simulink subsystem "VehicleEOMRef"  (R2025a)
settings: Solver=VariableStepAuto  StartTime=0.0  StopTime=10.0  RelTol=1e-3
undefined symbols (not defined in the file): Accel_bIi, AngularMomentum, AngularMomentumDot, Asensed_bIb, Forces, Moments, Omeg_BIb, Omeg_BIb_IC, OmegDtI_BIb, Pos_bii, Pos_bii_IC, Q_i2b, Q_i2b_IC, SimIn, SimPar, StateStruct, Vel_bEb_IC, Vel_bIi
libraries: starslibMathOperations x38, starslibAxisTransformations x25, starslibAirData x8, starslibKinematicalEquations x5, starslibGeodesy x4
(part 1 of 2)
settings Model: Creator=drhill  LastModifiedBy=alhallmark
settings SolverCC: AlgebraicLoopSolver=TrustRegion
settings OptimizationCC: ReuseModelBlockBuffer=off
settings DebuggingCC: UnconnectedInputMsg=warning  UnconnectedOutputMsg=warning  UnconnectedLineMsg=warning
settings ModelReferenceCC: EnableRefExpFcnMdlSchedulingChecks=on
settings RTWCC: GPUComputeCapability=3.5  DLArmComputeVersion=19.05

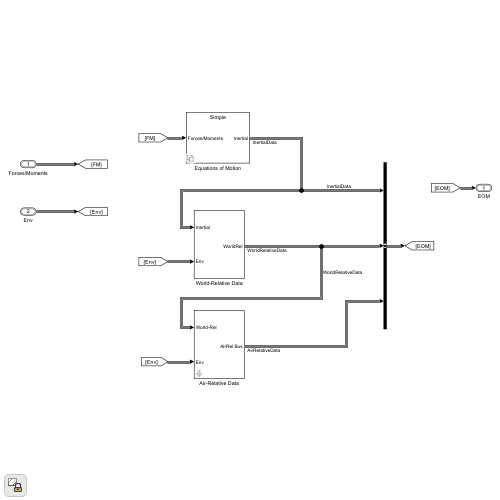
[thumbnail: Simulink's stored preview of the top-level diagram]
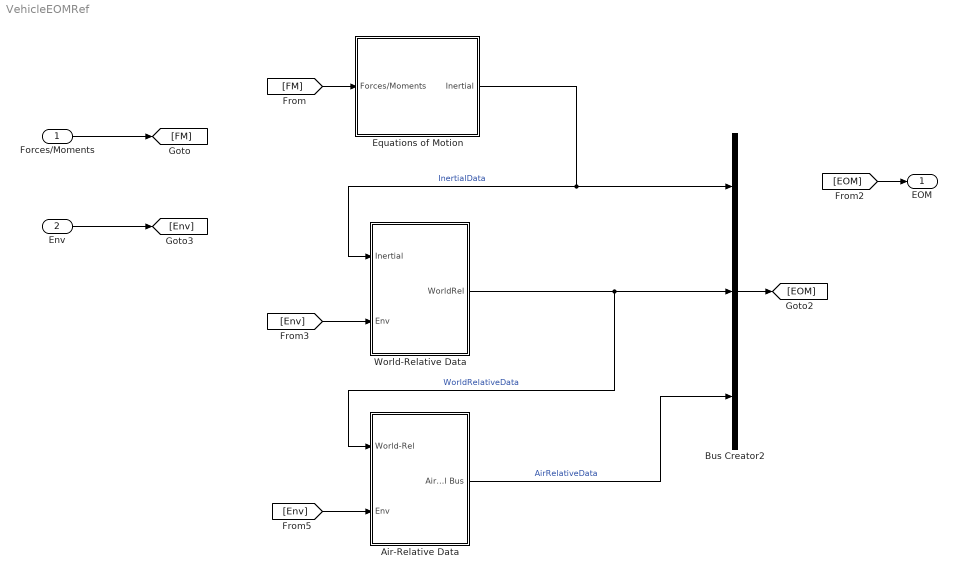
== system VehicleEOMRef ==
  Forces/Moments : Inport  OutDataTypeStr=Bus: ForceMomentBus
  Env : Inport  Port=2  OutDataTypeStr=Bus: EnvironmentBus
  Air-Relative Data : Subsystem  mask(Air-Relative Data (template)){}
      mask help: Template for common air-relative data.
  Bus Creator2 : BusCreator  Inputs=3  OutDataTypeStr=Bus: EomBus
  Equations of Motion : Subsystem  Variant=on  VariantControl=Variant1
  World-Relative Data : Subsystem
  EOM : Outport  OutDataTypeStr=Bus: EomBus
  wires:
  Forces/Moments/1 -> [FM]
  [FM] -> Equations of Motion/1(Forces/Moments)
  Bus Creator2/1 -> [EOM]
  [EOM] -> EOM/1
  Env/1 -> [Env]
  [Env] -> World-Relative Data/2(Env)
  [Env] -> Air-Relative Data/2(Env)
  Air-Relative Data/1(AirRel Bus) -> Bus Creator2/3  "AirRelativeData"
  Equations of Motion/1(Inertial) -> Bus Creator2/1, World-Relative Data/1(Inertial)  "InertialData"
  World-Relative Data/1(WorldRel) -> Air-Relative Data/1(World-Rel), Bus Creator2/2  "WorldRelativeData"

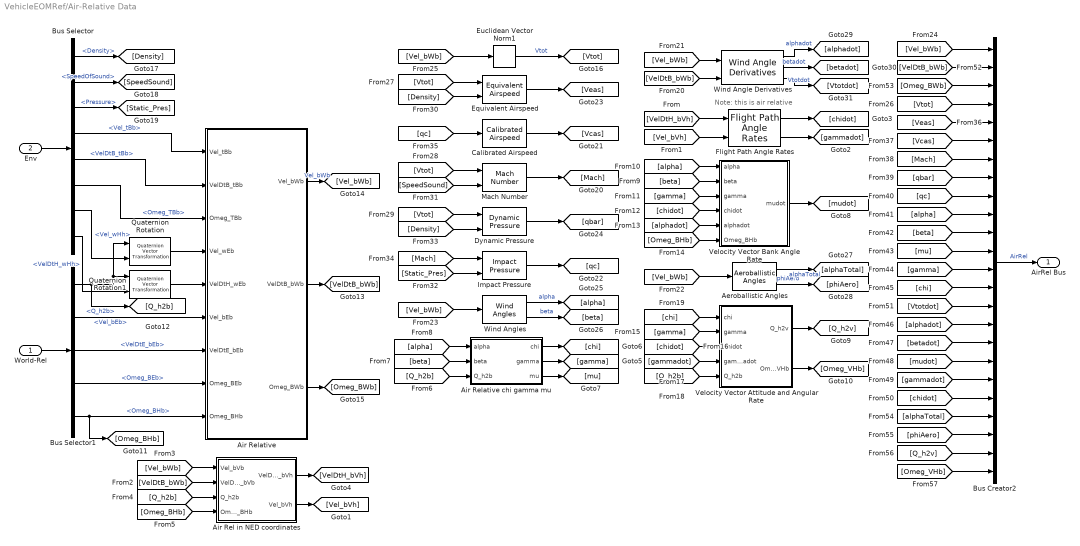
== system VehicleEOMRef/Air-Relative Data ==
  note: Note: this is air relative
  World-Rel : Inport
  Env : Inport  Port=2
  Aeroballistic Angles : starslibAirData/Aeroballistic Angles
  Air Rel in NED coordinates : Subsystem
  Air Relative : Subsystem
  Air Relative chi gamma mu : Subsystem
  Bus Creator2 : BusCreator  Inputs=24  OutDataTypeStr=Bus: AirRelBus
  Bus Selector : BusSelector  OutputSignals=Atmosphere.Density,Atmosphere.SpeedOfSound,Atmosphere.Pressure,Turbulence.Vel_tBb,Turbulence.VelDtB_tBb,Turbulence.Omeg_TBb,Wind.Vel_wHh,Wind.VelDtH_wHh
  Bus Selector1 : BusSelector  OutputSignals=Q_h2b,Vel_bEb,VelDtE_bEb,Omeg_BEb,Omeg_BHb
  Calibrated Airspeed : starslibAirData/Calibrated Airspeed  rhoref=SimIn.Environment.Atmos.rho0  Pref=SimIn.Environment.Atmos.Ps0  gamma=SimIn.Environment.Atmos.gamma
  Dynamic Pressure : starslibAirData/Dynamic Pressure
  Equivalent Airspeed : starslibAirData/Equivalent Airspeed  rhoref=SimIn.Environment.Atmos.rho0
  Euclidean Vector Norm1 : starslibMathOperations/Euclidean Vector Norm  dim=1
  Flight Path Angle Rates : starslibKinematicalEquations/Flight Path Angle Rates
  Impact Pressure : starslibAirData/Impact Pressure  gamma=SimIn.Environment.Atmos.gamma
  Mach Number : starslibAirData/Mach Number
  Quaternion Rotation : starslibAxisTransformations/Quaternion Vector Transformation  n=0
  Quaternion Rotation1 : starslibAxisTransformations/Quaternion Vector Transformation  n=0
  Velocity Vector Attitude and Angular Rate : Subsystem
  Velocity Vector Bank Angle Rate : Subsystem
  Wind Angle Derivatives : starslibAirData/Wind Angle Derivatives
  Wind Angles : starslibAirData/Wind Angles
  AirRel Bus : Outport
  wires:
  [Omeg_VHb] -> Bus Creator2/24
  [Q_h2v] -> Bus Creator2/23
  [phiAero] -> Bus Creator2/22
  [alphaTotal] -> Bus Creator2/21
  [Omeg_BWb] -> Bus Creator2/3
  [VelDtB_bWb] -> Bus Creator2/2
  [Vtotdot] -> Bus Creator2/15
  [chidot] -> Bus Creator2/20
  [gammadot] -> Bus Creator2/19
  [mudot] -> Bus Creator2/18
  [betadot] -> Bus Creator2/17
  [alphadot] -> Bus Creator2/16
  [chi] -> Bus Creator2/14
  [gamma] -> Bus Creator2/13
  [mu] -> Bus Creator2/12
  [beta] -> Bus Creator2/11
  [alpha] -> Bus Creator2/10
  [qc] -> Bus Creator2/9
  [qbar] -> Bus Creator2/8
  [Mach] -> Bus Creator2/7
  [Vcas] -> Bus Creator2/6
  [Veas] -> Bus Creator2/5
  Wind Angle Derivatives/3 -> [Vtotdot]  "Vtotdot"
  Wind Angle Derivatives/2 -> [betadot]  "betadot"
  Wind Angle Derivatives/1 -> [alphadot]  "alphadot"
  Aeroballistic Angles/2 -> [phiAero]  "phiAero"
  Aeroballistic Angles/1 -> [alphaTotal]  "alphaTotal"
  Wind Angles/2 -> [beta]  "beta"
  Wind Angles/1 -> [alpha]  "alpha"
  [qc] -> Calibrated Airspeed/1
  Calibrated Airspeed/1 -> [Vcas]
  [Mach] -> Impact Pressure/1
  Mach Number/1 -> [Mach]
  [Density] -> Dynamic Pressure/2
  [Density] -> Equivalent Airspeed/2
  [SpeedSound] -> Mach Number/2
  [Static_Pres] -> Impact Pressure/2
  [Vtot] -> Dynamic Pressure/1
  [Vtot] -> Mach Number/1
  [Vtot] -> Equivalent Airspeed/1
  Euclidean Vector Norm1/1 -> [Vtot]  "Vtot"
  Air Relative/3(Omeg_BWb) -> [Omeg_BWb]
  [Vel_bWb] -> Euclidean Vector Norm1/1
  [Vel_bWb] -> Bus Creator2/1
  [Vel_bWb] -> Wind Angles/1
  [Vel_bWb] -> Aeroballistic Angles/1
  [VelDtB_bWb] -> Wind Angle Derivatives/2
  [Vel_bWb] -> Wind Angle Derivatives/1
  Velocity Vector Attitude and Angular Rate/2(Omeg_VHb) -> [Omeg_VHb]
  Velocity Vector Attitude and Angular Rate/1(Q_h2v) -> [Q_h2v]
  [chi] -> Velocity Vector Attitude and Angular Rate/1(chi)
  [gammadot] -> Velocity Vector Attitude and Angular Rate/4(gammadot)
  [gamma] -> Velocity Vector Attitude and Angular Rate/2(gamma)
  [chidot] -> Velocity Vector Attitude and Angular Rate/3(" chidot")
  [Q_h2b] -> Velocity Vector Attitude and Angular Rate/5(Q_h2b)
  [Omeg_BHb] -> Velocity Vector Bank Angle Rate/6(Omeg_BHb)
  [alphadot] -> Velocity Vector Bank Angle Rate/5(alphadot)
  [chidot] -> Velocity Vector Bank Angle Rate/4(chidot)
  [gamma] -> Velocity Vector Bank Angle Rate/3(gamma)
  [alpha] -> Velocity Vector Bank Angle Rate/1(alpha)
  [beta] -> Velocity Vector Bank Angle Rate/2(beta)
  Velocity Vector Bank Angle Rate/1(mudot) -> [mudot]
  [alpha] -> Air Relative chi gamma mu/1(alpha)
  [beta] -> Air Relative chi gamma mu/2(beta)
  Air Relative chi gamma mu/3(mu) -> [mu]
  Air Relative chi gamma mu/2(gamma) -> [gamma]
  Air Relative chi gamma mu/1(chi) -> [chi]
  [Q_h2b] -> Air Relative chi gamma mu/3(Q_h2b)
  [Omeg_BHb] -> Air Rel in NED coordinates/4(Omeg_BHb)
  [Q_h2b] -> Air Rel in NED coordinates/3(Q_h2b)
  [Vel_bWb] -> Air Rel in NED coordinates/1(Vel_bVb)
  [VelDtB_bWb] -> Air Rel in NED coordinates/2(VelDtB_bVb)
  Air Rel in NED coordinates/2(Vel_bVh) -> [Vel_bVh]
  Air Rel in NED coordinates/1(VelDtH_bVh) -> [VelDtH_bVh]
  [Vel_bVh] -> Flight Path Angle Rates/2
  [VelDtH_bVh] -> Flight Path Angle Rates/1
  Flight Path Angle Rates/2 -> [gammadot]
  Flight Path Angle Rates/1 -> [chidot]
  Bus Selector/6 -> Air Relative/3(Omeg_TBb)  "<Omeg_TBb>"
  Bus Selector/5 -> Air Relative/2(VelDtB_tBb)  "<VelDtB_tBb>"
  Bus Selector/4 -> Air Relative/1(Vel_tBb)  "<Vel_tBb>"
  Bus Selector1/5 -> Air Relative/9(Omeg_BHb), [Omeg_BHb]  "<Omeg_BHb>"
  Bus Selector1/4 -> Air Relative/8(Omeg_BEb)  "<Omeg_BEb>"
  Bus Selector/3 -> [Static_Pres]  "<Pressure>"
  Bus Creator2/1 -> AirRel Bus/1  "AirRel"
  Equivalent Airspeed/1 -> [Veas]
  Impact Pressure/1 -> [qc]
  Quaternion Rotation1/1 -> Air Relative/5(VelDtH_wEb)
  Quaternion Rotation/1 -> Air Relative/4(Vel_wEb)
  Bus Selector1/3 -> Air Relative/7(VelDtE_bEb)  "<VelDtE_bEb>"
  Bus Selector1/2 -> Air Relative/6(Vel_bEb)  "<Vel_bEb>"
  Bus Selector1/1 -> [Q_h2b], Quaternion Rotation1/1, Quaternion Rotation/1  "<Q_h2b>"
  Bus Selector/8 -> Quaternion Rotation1/2  "<VelDtH_wHh>"
  Bus Selector/7 -> Quaternion Rotation/2  "<Vel_wHh>"
  Air Relative/2(VelDtB_bWb) -> [VelDtB_bWb]
  Dynamic Pressure/1 -> [qbar]
  Air Relative/1(Vel_bWb) -> [Vel_bWb]  "Vel_bWb"
  Bus Selector/1 -> [Density]  "<Density>"
  Bus Selector/2 -> [SpeedSound]  "<SpeedOfSound>"
  Env/1 -> Bus Selector/1
  World-Rel/1 -> Bus Selector1/1
  [Vtot] -> Bus Creator2/4

== system VehicleEOMRef/Equations of Motion ==
  Forces/Moments : Inport
  STARS : Subsystem  VariantControl=GVS_EOM_TYPE_LIMITED
  Simple : Subsystem  VariantControl=GVS_EOM_TYPE_SIMPLE
  Inertial : Outport

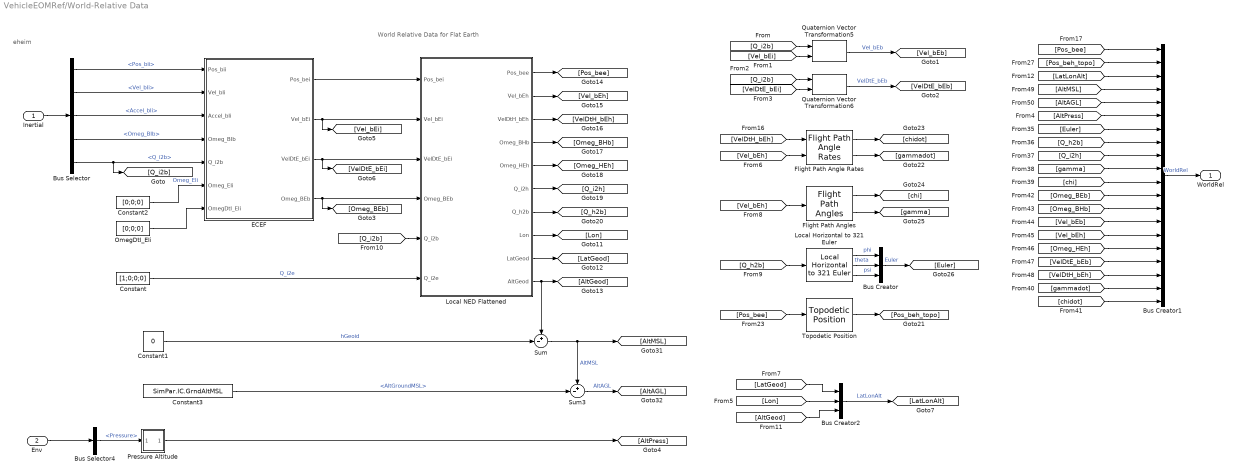
== system VehicleEOMRef/World-Relative Data ==
  note: World Relative Data for Flat Earth
  note: eheim
  Inertial : Inport
  Env : Inport  Port=2
  Bus Creator : BusCreator  Inputs=3  OutDataTypeStr=Bus: EulerBus
  Bus Creator1 : BusCreator  Inputs=20  OutDataTypeStr=Bus: WorldRelBus
  Bus Creator2 : BusCreator  Inputs=3  OutDataTypeStr=Bus: LatLonAltBus
  Bus Selector : BusSelector  OutputSignals=Pos_bii,Vel_bIi,Accel_bIi,Omeg_BIb,Q_i2b
  Bus Selector4 : BusSelector  OutputSignals=Atmosphere.Pressure
  Constant : Constant  Value=[1;0;0;0]  VectorParams1D=off
  Constant1 : Constant  Value=0  VectorParams1D=off
  Constant2 : Constant  Value=[0;0;0]  VectorParams1D=off
  Constant3 : Constant  Value=SimPar.IC.GrndAltMSL  VectorParams1D=off
  ECEF : Subsystem
  Flight Path Angle Rates : starslibKinematicalEquations/Flight Path Angle Rates
  Flight Path Angles : starslibKinematicalEquations/Flight Path Angles
  Local Horizontal to 321 Euler : starslibKinematicalEquations/Local Horizontal to 321 Euler
  Local NED Flattened : Subsystem
  OmegDtI_EIi : Constant  Value=[0;0;0]  VectorParams1D=off
  Pressure Altitude : Subsystem  mask(Pressure Alitude){standard=U.S. Naval Test Pilot School, u=SimIn.Units}
      mask prompts: standard "Select Standard"; u "STARS Units Structure"
      mask help:
      | Computes the standard day pressure alitude derived from the hydro static equation using parameters from one of the following sources:
      |  1) U.S. Standard Atmosphere, 1976
      |     Derived from Eqn 33a.
      |  2) National Oceanic and Atmospheric Administration
      |     http://www.srh.noaa.gov/images/epz/wxcalc/pressureAltitude.pdf
      |  3) U.S. Naval Test Pilot School
      |     USNTPS-FTM-NO. 108, Eqn 2.89
      mask init:
      | switch standard
      |     case 'U.S. Standard Atmosphere, 1976'
      |         UP = 1/u.Pa;
      |         KP = 1/1.01325e5;
      |         EP = (6.5/1000*8.31432e3/(9.80665*28.9644));
      |         KA = 288.15/(6.5/1000);
      |         UA = u.m;
      |     case 'National Oceanic and Atmospheric Administration'
      |         UP = 1/u.mbar;
      |         KP = 1/1013.25;
      |         EP = 0.190284;
      |         KA = 145366.45;
      |         UA = u.ft;
      |     case 'U.S. Naval Test Pilot School'
      |         UP = 1/u.psf;
      |         KP = 1/2116.217;
      |         EP = (32.17*0.0019812*96.93/32.174049);
      |         KA = 288.15/0.0019812;
      |         UA = u.ft;
      |     otherwise 
      |         error('Standard not valid')
      | end
      mask TypeOptions standard: U.S. Standard Atmosphere, 1976 | National Oceanic and Atmospheric Administration | U.S. Naval Test Pilot School
      mask Display:
      | port_label('input',1,'P')
      | port_label('output',1,'h')
  Quaternion Vector Transformation5 : starslibAxisTransformations/Quaternion Vector Transformation  n=0
  Quaternion Vector Transformation6 : starslibAxisTransformations/Quaternion Vector Transformation  n=0
  Sum : Sum  Inputs=+-|
  Sum3 : Sum  Inputs=+-|
  Topodetic Position : starslibGeodesy/Topodetic Position  Pos_bee=SimIn.EOM.Pos_bee  Q_e2h=SimIn.EOM.Q_e2h
  WorldRel : Outport
  wires:
  [chidot] -> Bus Creator1/20
  [gammadot] -> Bus Creator1/19
  [VelDtH_bEh] -> Bus Creator1/18
  [VelDtE_bEb] -> Bus Creator1/17
  [Omeg_HEh] -> Bus Creator1/16
  [Vel_bEh] -> Bus Creator1/15
  [Vel_bEb] -> Bus Creator1/14
  [Omeg_BHb] -> Bus Creator1/13
  [Omeg_BEb] -> Bus Creator1/12
  [chi] -> Bus Creator1/11
  [gamma] -> Bus Creator1/10
  [Q_i2h] -> Bus Creator1/9
  [Q_h2b] -> Bus Creator1/8
  [Euler] -> Bus Creator1/7
  [LatLonAlt] -> Bus Creator1/3
  [Pos_beh_topo] -> Bus Creator1/2
  [Pos_bee] -> Bus Creator1/1
  [AltPress] -> Bus Creator1/6
  [AltAGL] -> Bus Creator1/5
  [AltMSL] -> Bus Creator1/4
  Bus Creator2/1 -> [LatLonAlt]  "LatLonAlt"
  [AltGeod] -> Bus Creator2/3
  [LatGeod] -> Bus Creator2/1
  [Lon] -> Bus Creator2/2
  Pressure Altitude/1(Pressure Altitude MSL) -> [AltPress]
  Bus Selector4/1 -> Pressure Altitude/1(Static Pressure)  "<Pressure>"
  Env/1 -> Bus Selector4/1
  Inertial/1 -> Bus Selector/1
  Bus Creator/1 -> [Euler]  "Euler"
  Local Horizontal to 321 Euler/1 -> Bus Creator/1  "phi"
  Local Horizontal to 321 Euler/2 -> Bus Creator/2  "theta"
  Local Horizontal to 321 Euler/3 -> Bus Creator/3  "psi"
  [Q_i2b] -> Quaternion Vector Transformation5/1
  [Vel_bEi] -> Quaternion Vector Transformation5/2
  Quaternion Vector Transformation5/1 -> [Vel_bEb]  "Vel_bEb"
  [Q_i2b] -> Quaternion Vector Transformation6/1
  [VelDtE_bEi] -> Quaternion Vector Transformation6/2
  Quaternion Vector Transformation6/1 -> [VelDtE_bEb]  "VelDtE_bEb"
  Sum/1 -> Sum3/1, [AltMSL]  "AltMSL"
  Sum3/1 -> [AltAGL]  "AltAGL"
  Constant3/1 -> Sum3/2  "<AltGroundMSL>"
  [Vel_bEh] -> Flight Path Angle Rates/2
  [Vel_bEh] -> Flight Path Angles/1
  [Q_h2b] -> Local Horizontal to 321 Euler/1
  ECEF/2(Vel_bEi) -> [Vel_bEi], Local NED Flattened/2(Vel_bEi)
  ECEF/3("VelDtE_bEi ") -> [VelDtE_bEi], Local NED Flattened/3(VelDtE_bEi)
  ECEF/4(Omeg_BEb) -> [Omeg_BEb], Local NED Flattened/4(Omeg_BEb)
  [Q_i2b] -> Local NED Flattened/5(Q_i2b)
  Bus Selector/1 -> ECEF/1(Pos_bii)  "<Pos_bii>"
  Bus Selector/2 -> ECEF/2(Vel_bIi)  "<Vel_bIi>"
  Bus Selector/3 -> ECEF/3(Accel_bIi)  "<Accel_bIi>"
  Bus Selector/4 -> ECEF/4(Omeg_BIb)  "<Omeg_BIb>"
  Bus Selector/5 -> [Q_i2b], ECEF/5(Q_i2b)  "<Q_i2b>"
  OmegDtI_EIi/1 -> ECEF/7(OmegDtI_EIi)
  [Pos_bee] -> Topodetic Position/1
  Local NED Flattened/2(Vel_bEh) -> [Vel_bEh]
  Local NED Flattened/3(VelDtH_bEh) -> [VelDtH_bEh]
  Local NED Flattened/4(Omeg_BHb) -> [Omeg_BHb]
  Local NED Flattened/5(Omeg_HEh) -> [Omeg_HEh]
  Local NED Flattened/6(Q_i2h) -> [Q_i2h]
  Local NED Flattened/7(Q_h2b) -> [Q_h2b]
  [VelDtH_bEh] -> Flight Path Angle Rates/1
  Bus Creator1/1 -> WorldRel/1  "WorldRel"
  Topodetic Position/1 -> [Pos_beh_topo]
  Flight Path Angle Rates/1 -> [chidot]
  Flight Path Angle Rates/2 -> [gammadot]
  Flight Path Angles/1 -> [chi]
  Flight Path Angles/2 -> [gamma]
  ECEF/1(Pos_bei) -> Local NED Flattened/1(Pos_bei)
  Local NED Flattened/1(Pos_bee) -> [Pos_bee]
  Local NED Flattened/8(Lon) -> [Lon]
  Local NED Flattened/9(LatGeod) -> [LatGeod]
  Local NED Flattened/10(AltGeod) -> [AltGeod], Sum/1
  Constant2/1 -> ECEF/6(Omeg_EIi)  "Omeg_EIi"
  Constant/1 -> Local NED Flattened/6(Q_i2e)  "Q_i2e"
  Constant1/1 -> Sum/2  "hGeoid"

== system VehicleEOMRef/Air-Relative Data/Air Rel in NED coordinates ==
  note: eheim
      | bbacon
  note: Air relative velocity and acceleration as observed from the NED frame in NED coordinates.
  Vel_bVb : Inport
  VelDtB_bVb : Inport  Port=2
  Q_h2b : Inport  Port=3
  Omeg_BHb : Inport  Port=4
  Cross Product2 : starslibMathOperations/Cross Product
  Quaternion Conjugate2 : starslibMathOperations/Quaternion Conjugate  n=0
  Quaternion Rotation2 : starslibAxisTransformations/Quaternion Vector Transformation  n=0
  Quaternion Rotation3 : starslibAxisTransformations/Quaternion Vector Transformation  n=0
  Sum : Sum  Inputs=|++
  VelDtH_bVh : Outport
  Vel_bVh : Outport  Port=2
  wires:
  VelDtB_bVb/1 -> Sum/1
  Omeg_BHb/1 -> Cross Product2/1
  Quaternion Rotation3/1 -> VelDtH_bVh/1  "VelDtH_bVh"
  Sum/1 -> Quaternion Rotation3/2  "VelDtH_bVb"
  Cross Product2/1 -> Sum/2
  Vel_bVb/1 -> Cross Product2/2, Quaternion Rotation2/2
  Quaternion Conjugate2/1 -> Quaternion Rotation3/1, Quaternion Rotation2/1  "Q_b2h"
  Quaternion Rotation2/1 -> Vel_bVh/1  "Vel_bVh"
  Q_h2b/1 -> Quaternion Conjugate2/1

== system VehicleEOMRef/Air-Relative Data/Air Relative ==
  note: Assumes turbulence is subtractive.
  note: Air-Relative Vehicle States
  note: eheim
      | bbacon
  note: Vel_bWb = V_bEb - Vel_wEb - Vel_tBb
      | VelDtB_bWb = (VelDtE_bEb - Omeg_BEb x Vel_bEb) - (VelDtH_wEb - Omeg_BHb x Vel_wEb) - VelDtB_tBb
      | Omeg_BWb = Omeg_BHb - Omeg_TBb
  Vel_tBb : Inport
  VelDtB_tBb : Inport  Port=2
  Omeg_TBb : Inport  Port=3
  Vel_wEb : Inport  Port=4
  VelDtH_wEb : Inport  Port=5
  Vel_bEb : Inport  Port=6
  VelDtE_bEb : Inport  Port=7
  Omeg_BEb : Inport  Port=8
  Omeg_BHb : Inport  Port=9
  Cross Product1 : starslibMathOperations/Cross Product
  Cross Product2 : starslibMathOperations/Cross Product
  Sum1 : Sum  Inputs=+-|
  Sum2 : Sum  Inputs=+--
  Sum5 : Sum  Inputs=+--
  Sum6 : Sum  Inputs=|-+
  Sum7 : Sum  Inputs=+-|
  Vel_bWb : Outport
  VelDtB_bWb : Outport  Port=2
  Omeg_BWb : Outport  Port=3
  wires:
  VelDtB_tBb/1 -> Sum2/2
  Vel_tBb/1 -> Sum5/2
  Omeg_TBb/1 -> Sum1/2
  Sum1/1 -> Omeg_BWb/1  "Omeg_BWb"
  Omeg_BHb/1 -> Cross Product2/1, Sum1/1
  Vel_bEb/1 -> Sum5/1, Cross Product1/2
  Vel_wEb/1 -> Sum5/3, Cross Product2/2
  Sum5/1 -> Vel_bWb/1  "Vel_bWb"
  Omeg_BEb/1 -> Cross Product1/1
  VelDtE_bEb/1 -> Sum7/1
  Cross Product1/1 -> Sum7/2
  Cross Product2/1 -> Sum6/1
  VelDtH_wEb/1 -> Sum6/2
  Sum7/1 -> Sum2/1  "VelDtB_bEb"
  Sum6/1 -> Sum2/3  "VelDtB_wEb"
  Sum2/1 -> VelDtB_bWb/1  "VelDtB_bWb"

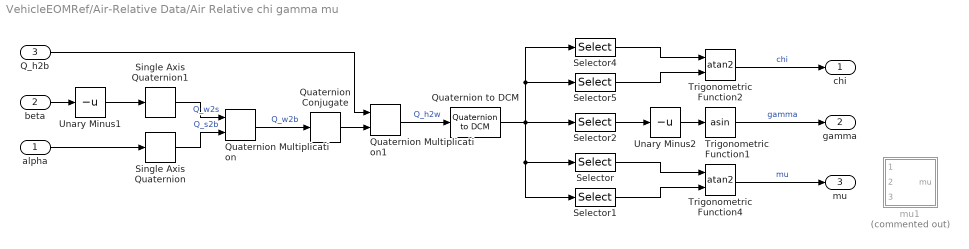
== system VehicleEOMRef/Air-Relative Data/Air Relative chi gamma mu ==
  alpha : Inport
  beta : Inport  Port=2
  Q_h2b : Inport  Port=3
  Quaternion Conjugate : starslibMathOperations/Quaternion Conjugate  n=0
  Quaternion Multiplication : starslibMathOperations/Quaternion Multiplication  n=0
  Quaternion Multiplication1 : starslibMathOperations/Quaternion Multiplication  n=0
  Quaternion to DCM : starslibAxisTransformations/Quaternion to DCM  n=0
  Selector : Selector  NumberOfDimensions=2  InputPortWidth=9  IndexOptions=Index vector (dialog),Index vector (dialog)  Indices=2,3  OutputSizes=1,1
  Selector1 : Selector  NumberOfDimensions=2  InputPortWidth=9  IndexOptions=Index vector (dialog),Index vector (dialog)  Indices=3,3  OutputSizes=1,1
  Selector2 : Selector  NumberOfDimensions=2  InputPortWidth=9  IndexOptions=Index vector (dialog),Index vector (dialog)  Indices=1,3  OutputSizes=1,1
  Selector4 : Selector  NumberOfDimensions=2  InputPortWidth=9  IndexOptions=Index vector (dialog),Index vector (dialog)  Indices=1,2  OutputSizes=1,1
  Selector5 : Selector  NumberOfDimensions=2  InputPortWidth=9  IndexOptions=Index vector (dialog),Index vector (dialog)  Indices=1,1  OutputSizes=1,1
  Single Axis Quaternion : starslibAxisTransformations/Single Axis Quaternion  RotAxis=y  n=0
  Single Axis Quaternion1 : starslibAxisTransformations/Single Axis Quaternion  RotAxis=z  n=0
  Trigonometric Function1 : Trigonometry  Operator=asin
  Trigonometric Function2 : Trigonometry  Operator=atan2
  Trigonometric Function4 : Trigonometry  Operator=atan2
  Unary Minus1 : UnaryMinus
  Unary Minus2 : UnaryMinus
  mu1 : Subsystem  Commented=on
  chi : Outport
  gamma : Outport  Port=2
  mu : Outport  Port=3
  wires:
  Trigonometric Function2/1 -> chi/1  "chi"
  Single Axis Quaternion/1 -> Quaternion Multiplication/2  "Q_s2b"
  Unary Minus2/1 -> Trigonometric Function1/1
  Quaternion Conjugate/1 -> Quaternion Multiplication1/2
  Q_h2b/1 -> Quaternion Multiplication1/1
  alpha/1 -> Single Axis Quaternion/1
  Quaternion to DCM/1 -> Selector1/1, Selector/1, Selector4/1, Selector5/1, Selector2/1
  Trigonometric Function1/1 -> gamma/1  "gamma"
  Selector1/1 -> Trigonometric Function4/2
  Quaternion Multiplication/1 -> Quaternion Conjugate/1  "Q_w2b"
  Single Axis Quaternion1/1 -> Quaternion Multiplication/1  "Q_w2s"
  Unary Minus1/1 -> Single Axis Quaternion1/1
  Selector4/1 -> Trigonometric Function2/1
  Selector5/1 -> Trigonometric Function2/2
  Quaternion Multiplication1/1 -> Quaternion to DCM/1  "Q_h2w"
  beta/1 -> Unary Minus1/1
  Selector/1 -> Trigonometric Function4/1
  Trigonometric Function4/1 -> mu/1  "mu"
  Selector2/1 -> Unary Minus2/1

== system VehicleEOMRef/Air-Relative Data/Velocity Vector Attitude and Angular Rate ==
  note: eheim
      | bbacon
  note: Note: this is air relative
  chi : Inport
  gamma : Inport  Port=2
  " chidot" : Inport  Port=3
  gammadot : Inport  Port=4
  Q_h2b : Inport  Port=5
  Angular Rate of Navigation from NED : starslibKinematicalEquations/Angular Rate of Navigation from NED
  Quaternion Conjugate1 : starslibMathOperations/Quaternion Conjugate  n=0
  Quaternion Multiplication1 : starslibMathOperations/Quaternion Multiplication  n=0
  Quaternion Multiplication2 : starslibMathOperations/Quaternion Multiplication  n=0
  Quaternion Rotation1 : starslibAxisTransformations/Quaternion Vector Transformation  n=0
  Single Axis Quaternion2 : starslibAxisTransformations/Single Axis Quaternion  RotAxis=y  n=0
  Single Axis Quaternion3 : starslibAxisTransformations/Single Axis Quaternion  RotAxis=z  n=0
  Q_h2v : Outport
  Omeg_VHb : Outport  Port=2
  wires:
  Q_h2b/1 -> Quaternion Multiplication2/2
  Quaternion Conjugate1/1 -> Quaternion Multiplication2/1  "Q_v2h"
  Quaternion Multiplication2/1 -> Quaternion Rotation1/1  "Q_v2b"
  Single Axis Quaternion2/1 -> Quaternion Multiplication1/2
  Single Axis Quaternion3/1 -> Quaternion Multiplication1/1
  Quaternion Multiplication1/1 -> Q_h2v/1, Quaternion Conjugate1/1  "Q_h2v"
  chi/1 -> Single Axis Quaternion3/1
  gamma/1 -> Single Axis Quaternion2/1, Angular Rate of Navigation from NED/1
  gammadot/1 -> Angular Rate of Navigation from NED/3
  " chidot"/1 -> Angular Rate of Navigation from NED/2
  Angular Rate of Navigation from NED/1 -> Quaternion Rotation1/2  "Omeg_VHv"
  Quaternion Rotation1/1 -> Omeg_VHb/1  "Omeg_VHb"

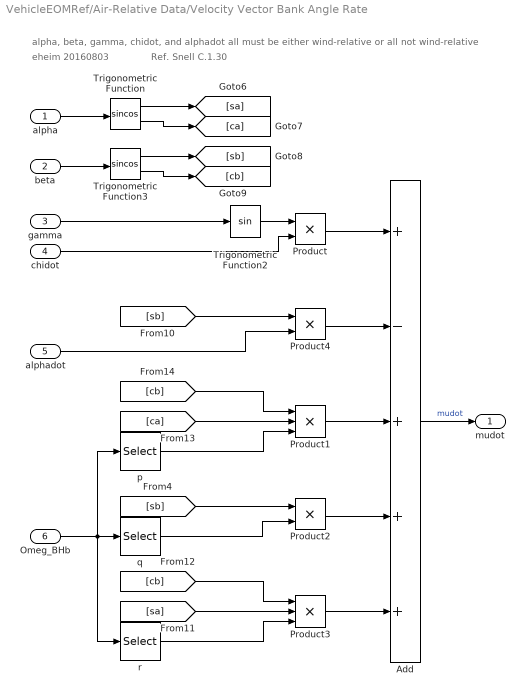
== system VehicleEOMRef/Air-Relative Data/Velocity Vector Bank Angle Rate ==
  note: Ref. Snell C.1.30
  note: eheim 20160803
  note: alpha, beta, gamma, chidot, and alphadot all must be either wind-relative or all not wind-relative
  alpha : Inport
  beta : Inport  Port=2
  gamma : Inport  Port=3
  chidot : Inport  Port=4
  alphadot : Inport  Port=5
  Omeg_BHb : Inport  Port=6
  Add : Sum  Inputs=+-+++
  Product : Product
  Product1 : Product  Inputs=3
  Product2 : Product
  Product3 : Product  Inputs=3
  Product4 : Product
  Trigonometric Function : Trigonometry  Operator=sincos
  Trigonometric Function2 : Trigonometry
  Trigonometric Function3 : Trigonometry  Operator=sincos
  p : Selector  NumberOfDimensions=2  InputPortWidth=3  IndexOptions=Index vector (dialog),Index vector (dialog)  Indices=1,1  OutputSizes=1,1
  q : Selector  NumberOfDimensions=2  InputPortWidth=3  IndexOptions=Index vector (dialog),Index vector (dialog)  Indices=2,1  OutputSizes=1,1
  r : Selector  NumberOfDimensions=2  InputPortWidth=3  IndexOptions=Index vector (dialog),Index vector (dialog)  Indices=3,1  OutputSizes=1,1
  mudot : Outport
  wires:
  Omeg_BHb/1 -> p/1, q/1, r/1
  [sa] -> Product3/2
  Trigonometric Function2/1 -> Product/1
  gamma/1 -> Trigonometric Function2/1
  alphadot/1 -> Product4/2
  [sb] -> Product2/1
  beta/1 -> Trigonometric Function3/1
  Trigonometric Function/1 -> [sa]
  Add/1 -> mudot/1  "mudot"
  r/1 -> Product3/3
  [sb] -> Product4/1
  q/1 -> Product2/2
  [cb] -> Product3/1
  Trigonometric Function3/2 -> [cb]
  alpha/1 -> Trigonometric Function/1
  Trigonometric Function3/1 -> [sb]
  p/1 -> Product1/3
  chidot/1 -> Product/2
  Product2/1 -> Add/4
  Product/1 -> Add/1
  Product3/1 -> Add/5
  Product4/1 -> Add/2
  Product1/1 -> Add/3
  [ca] -> Product1/2
  [cb] -> Product1/1
  Trigonometric Function/2 -> [ca]

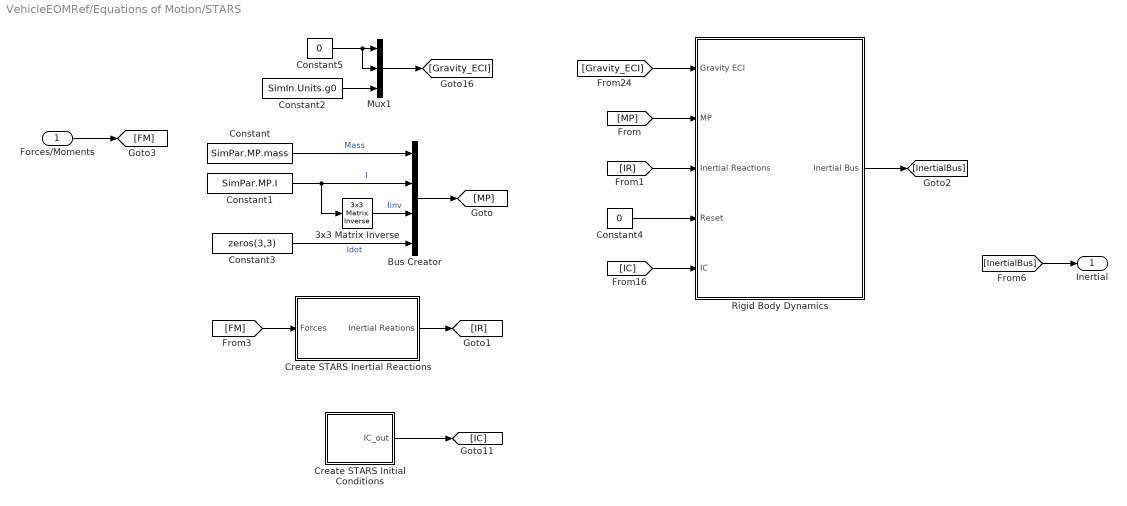
== system VehicleEOMRef/Equations of Motion/STARS ==
  Forces/Moments : Inport
  3x3 Matrix Inverse : starslibMathOperations/3x3 Matrix Inverse
  Bus Creator : BusCreator  Inputs=4
  Constant : Constant  Value=SimPar.MP.mass
  Constant1 : Constant  Value=SimPar.MP.I
  Constant2 : Constant  Value=SimIn.Units.g0
  Constant3 : Constant  Value=zeros(3,3)
  Constant4 : Constant  Value=0
  Constant5 : Constant  Value=0
  Create STARS Inertial Reactions : Subsystem
  Create STARS Initial Conditions : Subsystem
  Mux1 : Mux  Inputs=3
  Rigid Body Dynamics : Subsystem  mask(Rigid Body Dynamics){K_QuatStab=0.1, K_Idot=0, IC_Accels=off, Accel_i_IC=SimPar.EOM.Accel_bIi, ASensed_IC=SimPar.EOM.Asensed_bIb, OmegaDot_IC=SimPar.EOM.OmegDtI_BIb}
      mask prompts: K_QuatStab "Quaternion stability gain (k*dt <= 1)"; K_Idot "Varying inertia coefficient (0 to 1)"; IC_Accels "Set acceleration Initial Conditions (IC):"; Accel_i_IC "Inertial linear acceleration IC"; ASensed_IC "Sensed body axis linear acceleration IC"; OmegaDot_IC "Body axis angular acceleration IC"
      mask help: Rigid body equations of motion relative to an inertial frame.
  Inertial : Outport  OutDataTypeStr=Bus: InertialBus  VectorParamsAs1DForOutWhenUnconnected=off
  wires:
  [InertialBus] -> Inertial/1
  Rigid Body Dynamics/1(Inertial Bus) -> [InertialBus]
  [IR] -> Rigid Body Dynamics/3(Inertial Reactions)
  [MP] -> Rigid Body Dynamics/2(MP)
  Bus Creator/1 -> [MP]
  Constant/1 -> Bus Creator/1  "Mass"
  Constant1/1 -> 3x3 Matrix Inverse/1, Bus Creator/2  "I"
  Constant3/1 -> Bus Creator/4  "Idot"
  3x3 Matrix Inverse/1 -> Bus Creator/3  "Iinv"
  [IC] -> Rigid Body Dynamics/5(IC)
  Constant2/1 -> Mux1/3
  Constant5/1 -> Mux1/2, Mux1/1
  Mux1/1 -> [Gravity_ECI]
  [Gravity_ECI] -> Rigid Body Dynamics/1(Gravity ECI)
  Create STARS Initial Conditions/1(IC_out) -> [IC]
  Create STARS Inertial Reactions/1(Inertial Reations) -> [IR]
  Forces/Moments/1 -> [FM]
  [FM] -> Create STARS Inertial Reactions/1(Forces)
  Constant4/1 -> Rigid Body Dynamics/4(Reset)

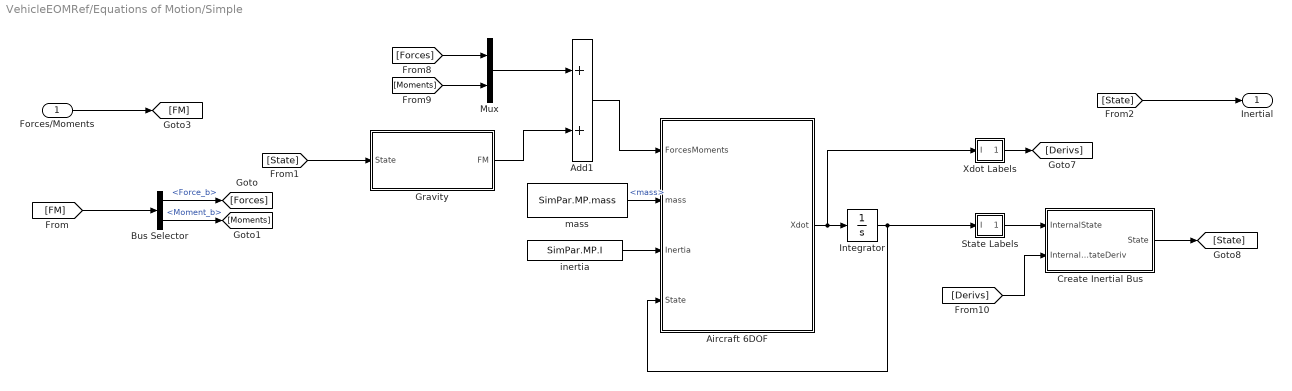
== system VehicleEOMRef/Equations of Motion/Simple ==
  Forces/Moments : Inport
  Add1 : Sum
  Aircraft 6DOF : Subsystem
  Bus Selector : BusSelector  OutputSignals=Total.Force_b,Total.Moment_b
  Create Inertial Bus : Subsystem
  Gravity : Subsystem
  Integrator : Integrator  InitialCondition=[SimPar.EOM.Vel_bEb; SimPar.EOM.Omeg_BIb; SimPar.EOM.Pos_bii; SimPar.EOM.Q_i2b]  LimitOutput=on  UpperSaturationLimit=[inf; inf; inf; 10; 10; 10; inf; inf; inf; 1; 1; 1; 1]  LowerSaturationLimit=-[inf; inf; inf; 10; 10; 10; inf; inf; inf; 1; 1; 1; 1]  ContinuousStateAttributes='EOMStates'
  Mux : Mux  Inputs=[3 3]
  State Labels : Subsystem
  Xdot Labels : Subsystem
  inertia : Constant  Value=SimPar.MP.I
  mass : Constant  Value=SimPar.MP.mass
  Inertial : Outport  OutDataTypeStr=Bus: InertialBus  VectorParamsAs1DForOutWhenUnconnected=off
  wires:
  Bus Selector/2 -> [Moments]  "<Moment_b>"
  Bus Selector/1 -> [Forces]  "<Force_b>"
  [FM] -> Bus Selector/1
  [State] -> Gravity/1(State)
  [Derivs] -> Create Inertial Bus/2(InternalStateDeriv)
  Create Inertial Bus/1(State) -> [State]
  State Labels/1(O) -> Create Inertial Bus/1(InternalState)
  Mux/1 -> Add1/1
  [Moments] -> Mux/2
  [Forces] -> Mux/1
  Gravity/1(FM) -> Add1/2
  inertia/1 -> Aircraft 6DOF/3(Inertia)
  Add1/1 -> Aircraft 6DOF/1(ForcesMoments)
  Integrator/1 -> Aircraft 6DOF/4(State), State Labels/1(I)
  Aircraft 6DOF/1(Xdot) -> Integrator/1, Xdot Labels/1(I)
  mass/1 -> Aircraft 6DOF/2(mass)  "<mass>"
  Xdot Labels/1(O) -> [Derivs]
  Forces/Moments/1 -> [FM]
  [State] -> Inertial/1

== system VehicleEOMRef/World-Relative Data/ECEF ==
  note: Pos_bii - Position of the body origin, b (center of mass) relative to the inertial origin, i (center of world) in inertial coordinates, i.
      | Vel_bIi - Inertial velocity of point b with respect to the inertial frame, I expressed in inertial coordinates, i.
      | Accel_bIi - Inertial acceleration of point b with respect to the inertial frame, I expressed in inertial coordinates, i.
      | Omeg_EIi  - Angular rate of the world frame, E with respect to the inertial frame, I in inertial coordinates, i.
      | Vel_bEi - Velocity of point, b with respect to the world frame, E expressed in inertial coordinates, i.
      | VelDtE_bEi - Acceleration of point, b as observed from the world frame, E and relative to the world frame, E expressed in inertial coordinates, i.
      | Omeg_BEb - Angular rate of the body frame with respect to the world frame, E expressed in body coordinates, b.
  note: World-relative velocity, acceleration, and angular rate
  note: eheim
      | bbacon
  note: Given:
      | 1..Origins of inertial frame and world frame are coincident, i.e. Pos_bei = Pos_bii
      | 2. World frame is not moving relative to the inertial frame, i.e. Vel_eIi = 0
      | 3. World frame is not accelerating relative to the inertial frame, i.e. VelDtI_eIi = 0
      | 4. Vel_bIi = Vel_eIi + Vel_bEi + Omeg_EIi x Pos_bei
      | 5. Accel_bIi = VelDtI_bIi
      |                     = VelDtI_eIi
      |                     + VelDtE_bEi
      |                     + OmegDtI_EIi x Pos_bei
      |                     + 2*Omeg_BEi x Vel_bEi
      |                     + Omeg_EIi x Omeg_EIi x Pos_bei
      |
      | Then:
      | Vel_bEi = Vel_bIi - Omeg_EIi x Pos_bii
      |
      | VelDtE_bEi  = VelDtI_bIi
      |                     - 2*Omeg_EIi x (Vel_bIi  - Omeg_EIi x Pos_bei)
      |                     - Omeg_EIi x Omeg_EIi x Pos_bei
      |
      |                     = VelDtI_bIi
      |                     - 2*Omeg_EIi x Vel_bIi
      |                     + Omega_EIi x Omeg_EIi x Pos_bei
  Pos_bii : Inport
  Vel_bIi : Inport  Port=2
  Accel_bIi : Inport  Port=3
  Omeg_BIb : Inport  Port=4
  Q_i2b : Inport  Port=5
  Omeg_EIi : Inport  Port=6
  OmegDtI_EIi : Inport  Port=7
  Add2 : Sum  Inputs=+--+
  Gain : Gain  Gain=2
  Quaternion Vector Transformation2 : starslibAxisTransformations/Quaternion Vector Transformation  n=0
  Subtract1 : Sum  Inputs=-+
  Subtract2 : Sum  Inputs=-+
  w x (w x r) : starslibMathOperations/Cross Product
  w x r : starslibMathOperations/Cross Product
  w x v : starslibMathOperations/Cross Product
  w x v1 : starslibMathOperations/Cross Product
  Pos_bei : Outport
  Vel_bEi : Outport  Port=2
  "VelDtE_bEi " : Outport  Port=3
  Omeg_BEb : Outport  Port=4
  wires:
  Subtract2/1 -> Omeg_BEb/1  "Omeg_BEb"
  Pos_bii/1 -> w x r/2, w x v1/2, Pos_bei/1
  Omeg_EIi/1 -> w x (w x r)/1, w x v/1, w x r/1, Quaternion Vector Transformation2/2
  Vel_bIi/1 -> w x v/2, Subtract1/2
  Add2/1 -> "VelDtE_bEi "/1  "VelDtE_bEi"
  Accel_bIi/1 -> Add2/1
  w x r/1 -> w x (w x r)/2, Subtract1/1
  w x (w x r)/1 -> Add2/4
  w x v/1 -> Gain/1
  Gain/1 -> Add2/3
  Quaternion Vector Transformation2/1 -> Subtract2/1
  Subtract1/1 -> Vel_bEi/1  "Vel_bEi"
  w x v1/1 -> Add2/2
  OmegDtI_EIi/1 -> w x v1/1
  Omeg_BIb/1 -> Subtract2/2
  Q_i2b/1 -> Quaternion Vector Transformation2/1

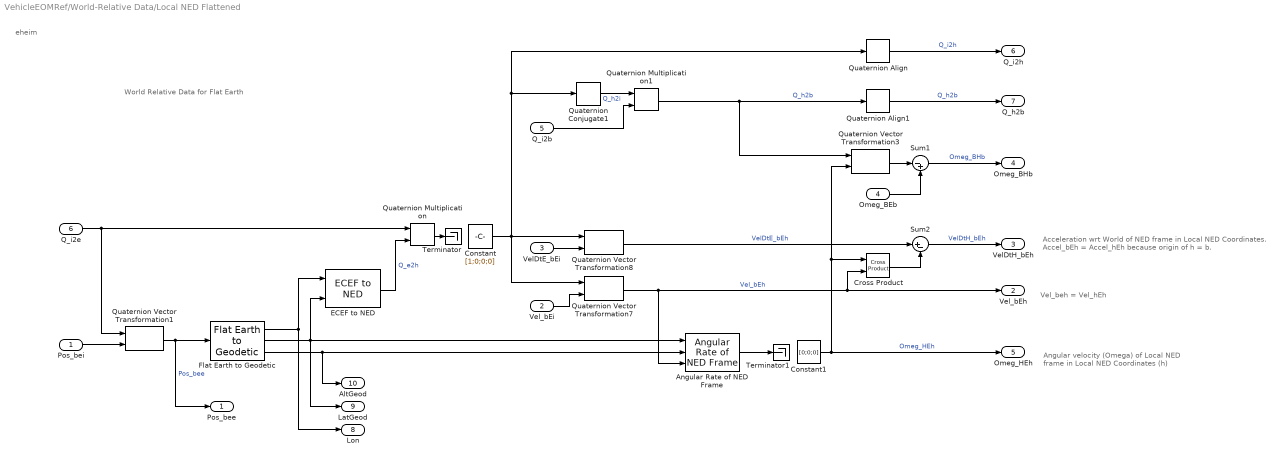
== system VehicleEOMRef/World-Relative Data/Local NED Flattened ==
  note: World Relative Data for Flat Earth
  note: Angular velocity (Omega) of Local
      | NED frame in Local NED Coordinates (h)
  note: Acceleration wrt World of NED frame in Local NED Coordinates.
      | Accel_bEh = Accel_hEh because origin of h = b.
  note: Vel_beh = Vel_hEh
  note: eheim
  Pos_bei : Inport
  Vel_bEi : Inport  Port=2
  VelDtE_bEi : Inport  Port=3
  Omeg_BEb : Inport  Port=4
  Q_i2b : Inport  Port=5
  Q_i2e : Inport  Port=6
  Angular Rate of NED Frame : starslibGeodesy/Angular Rate of NED Frame  a=SimIn.Environment.Earth.RadiusEquator  e=SimIn.Environment.Earth.Eccentricity
  Constant : Constant  Value=[1;0;0;0]  VectorParams1D=off
  Constant1 : Constant  Value=[0;0;0]  VectorParams1D=off
  Cross Product : starslibMathOperations/Cross Product
  ECEF to NED : starslibGeodesy/ECEF to NED
  Flat Earth to Geodetic : starslibGeodesy/Flat Earth to Geodetic  lat=SimIn.IC.LatGeod  lon=SimIn.IC.Lon  a=SimIn.Environment.Earth.RadiusEquator  e=SimIn.Environment.Earth.Eccentricity
  Quaternion Align : starslibMathOperations/Quaternion Align  n=0
  Quaternion Align1 : starslibMathOperations/Quaternion Align  n=0
  Quaternion Conjugate1 : starslibMathOperations/Quaternion Conjugate  n=0
  Quaternion Multiplication : starslibMathOperations/Quaternion Multiplication  n=0
  Quaternion Multiplication1 : starslibMathOperations/Quaternion Multiplication  n=0
  Quaternion Vector Transformation{1,3,7..8} (4 alike) : starslibAxisTransformations/Quaternion Vector Transformation  n=0
  Sum1 : Sum  Inputs=|-+
  Sum2 : Sum  Inputs=|+-
  Terminator : Terminator
  Terminator1 : Terminator
  Pos_bee : Outport  PortDimensions=[3,1]
  Vel_bEh : Outport  Port=2  PortDimensions=[3,1]
  VelDtH_bEh : Outport  Port=3  PortDimensions=[3,1]
  Omeg_BHb : Outport  Port=4  PortDimensions=[3,1]
  Omeg_HEh : Outport  Port=5  PortDimensions=[3,1]
  Q_i2h : Outport  Port=6  PortDimensions=[4,1]
  Q_h2b : Outport  Port=7  PortDimensions=[4,1]
  Lon : Outport  Port=8
  LatGeod : Outport  Port=9
  AltGeod : Outport  Port=10
  wires:
  Constant1/1 -> Quaternion Vector Transformation3/2, Cross Product/1, Omeg_HEh/1  "Omeg_HEh"
  Quaternion Vector Transformation3/1 -> Sum1/1
  Sum1/1 -> Omeg_BHb/1  "Omeg_BHb"
  Cross Product/1 -> Sum2/2
  Sum2/1 -> VelDtH_bEh/1  "VelDtH_bEh"
  Constant/1 -> Quaternion Vector Transformation7/1, Quaternion Vector Transformation8/1, Quaternion Conjugate1/1, Quaternion Align/1
  Quaternion Conjugate1/1 -> Quaternion Multiplication1/1  "Q_h2i"
  Quaternion Multiplication1/1 -> Quaternion Align1/1, Quaternion Vector Transformation3/1  "Q_h2b"
  Q_i2b/1 -> Quaternion Multiplication1/2
  Quaternion Align1/1 -> Q_h2b/1  "Q_h2b"
  Quaternion Align/1 -> Q_i2h/1  "Q_i2h"
  Vel_bEi/1 -> Quaternion Vector Transformation7/2
  Quaternion Vector Transformation7/1 -> Angular Rate of NED Frame/3, Cross Product/2, Vel_bEh/1  "Vel_bEh"
  VelDtE_bEi/1 -> Quaternion Vector Transformation8/2
  Quaternion Vector Transformation8/1 -> Sum2/1  "VelDtE_bEh"
  Omeg_BEb/1 -> Sum1/2
  Q_i2e/1 -> Quaternion Multiplication/1, Quaternion Vector Transformation1/1
  ECEF to NED/1 -> Quaternion Multiplication/2  "Q_e2h"
  Quaternion Vector Transformation1/1 -> Pos_bee/1, Flat Earth to Geodetic/1  "Pos_bee"
  Pos_bei/1 -> Quaternion Vector Transformation1/2
  Flat Earth to Geodetic/1 -> ECEF to NED/1, Lon/1
  Flat Earth to Geodetic/2 -> Angular Rate of NED Frame/1, ECEF to NED/2, LatGeod/1
  Flat Earth to Geodetic/3 -> Angular Rate of NED Frame/2, AltGeod/1
  Quaternion Multiplication/1 -> Terminator/1
  Angular Rate of NED Frame/1 -> Terminator1/1

== system VehicleEOMRef/World-Relative Data/Pressure Altitude ==
  Static Pressure : Inport
  Constant : Constant
  Convert Altitude Units : Gain  Gain=UA
  Convert Pressure Units : Gain  Gain=UP
  Exponent : Constant  Value=EP
  KA : Gain  Gain=KA
  KP : Gain  Gain=KP
  Math Function : Math  Operator=pow  SignedPower=on
  Subtract : Sum  Inputs=+-
  Pressure Altitude MSL : Outport
  wires:
  Exponent/1 -> Math Function/2
  Static Pressure/1 -> Convert Pressure Units/1
  Constant/1 -> Subtract/1
  Math Function/1 -> Subtract/2
  KA/1 -> Convert Altitude Units/1
  Convert Altitude Units/1 -> Pressure Altitude MSL/1  "AltPresMSL"
  Convert Pressure Units/1 -> KP/1
  KP/1 -> Math Function/1
  Subtract/1 -> KA/1

== system VehicleEOMRef/Air-Relative Data/Air Relative chi gamma mu/mu1 ==
  Q_h2v : Inport
  Q_h2b : Inport  Port=2
  Q_w2b : Inport  Port=3
  Gain : Gain  Gain=2
  Quaternion Align : starslibMathOperations/Quaternion Align  n=0
  Quaternion Conjugate : starslibMathOperations/Quaternion Conjugate  n=0
  Quaternion Conjugate1 : starslibMathOperations/Quaternion Conjugate  n=0
  Quaternion Multiplication2 : starslibMathOperations/Quaternion Multiplication  n=0
  Quaternion Multiplication3 : starslibMathOperations/Quaternion Multiplication  n=0
  Trigonometric Function1 : Trigonometry  Operator=atan2  OutputSignalType=real
  q1 : Selector  NumberOfDimensions=2  InputPortWidth=3  IndexOptions=Index vector (dialog),Select all  Indices=1,1  OutputSizes=1,1
  q2 : Selector  NumberOfDimensions=2  InputPortWidth=3  IndexOptions=Index vector (dialog),Select all  Indices=2,1  OutputSizes=1,1
  mu : Outport
  wires:
  q2/1 -> Trigonometric Function1/1
  q1/1 -> Trigonometric Function1/2
  Quaternion Multiplication2/1 -> Quaternion Multiplication3/1  "Q_v2b"
  Gain/1 -> mu/1  "mu"
  Quaternion Conjugate1/1 -> Quaternion Multiplication2/1  "Q_v2h"
  Trigonometric Function1/1 -> Gain/1
  Q_w2b/1 -> Quaternion Conjugate/1
  Quaternion Multiplication3/1 -> Quaternion Align/1  "Q_v2w"
  Quaternion Conjugate/1 -> Quaternion Multiplication3/2  "Q_b2w"
  Quaternion Align/1 -> q2/1, q1/1
  Q_h2v/1 -> Quaternion Conjugate1/1
  Q_h2b/1 -> Quaternion Multiplication2/2

== system VehicleEOMRef/Equations of Motion/STARS/Create STARS Inertial Reactions ==
  Forces : Inport
  Bus Assignment : BusAssignment  AssignedSignals=Forces,Moments,AngularMomentum,AngularMomentumDot
  Bus Selector : BusSelector  OutputSignals=Total.Force_b,Total.Moment_b,Total.H_b,Total.Hdot_b
  RenameInertialReactionsBus : Subsystem
  Inertial Reations : Outport  VectorParamsAs1DForOutWhenUnconnected=off
  wires:
  Bus Assignment/1 -> Inertial Reations/1
  [Hdot] -> Bus Assignment/5
  [H] -> Bus Assignment/4
  [Moments_b] -> Bus Assignment/3  "Moment_b"
  RenameInertialReactionsBus/1(IR) -> Bus Assignment/1
  [Forces_b] -> Bus Assignment/2  "Force_b"
  Bus Selector/4 -> [Hdot]  "<Hdot_b>"
  Bus Selector/3 -> [H]  "<H_b>"
  Bus Selector/2 -> [Moments_b]  "<Moment_b>"
  Bus Selector/1 -> [Forces_b]  "<Force_b>"
  [FM] -> Bus Selector/1
  Forces/1 -> [FM]

== system VehicleEOMRef/Equations of Motion/STARS/Create STARS Initial Conditions ==
  Bus Assignment : BusAssignment  AssignedSignals=Pos_bii_IC,Vel_bEb_IC,Q_i2b_IC,Omeg_BIb_IC
  Bus Selector : BusSelector  OutputSignals=Pos_bii,Vel_bEb,Q_i2b,Omeg_BIb
  RenameIcOutputBus : Subsystem
  IC_out : Outport  VectorParamsAs1DForOutWhenUnconnected=off
  wires:
  Bus Selector/4 -> Bus Assignment/5  "<Omeg_BIb>"
  Bus Selector/3 -> Bus Assignment/4  "<Q_i2b>"
  Bus Selector/2 -> Bus Assignment/3  "<Vel_bEb>"
  Bus Selector/1 -> Bus Assignment/2  "<Pos_bii>"
  RenameIcOutputBus/1(Out1) -> Bus Assignment/1
  Bus Assignment/1 -> IC_out/1  "IC_Out"
  [EOM_IC] -> Bus Selector/1

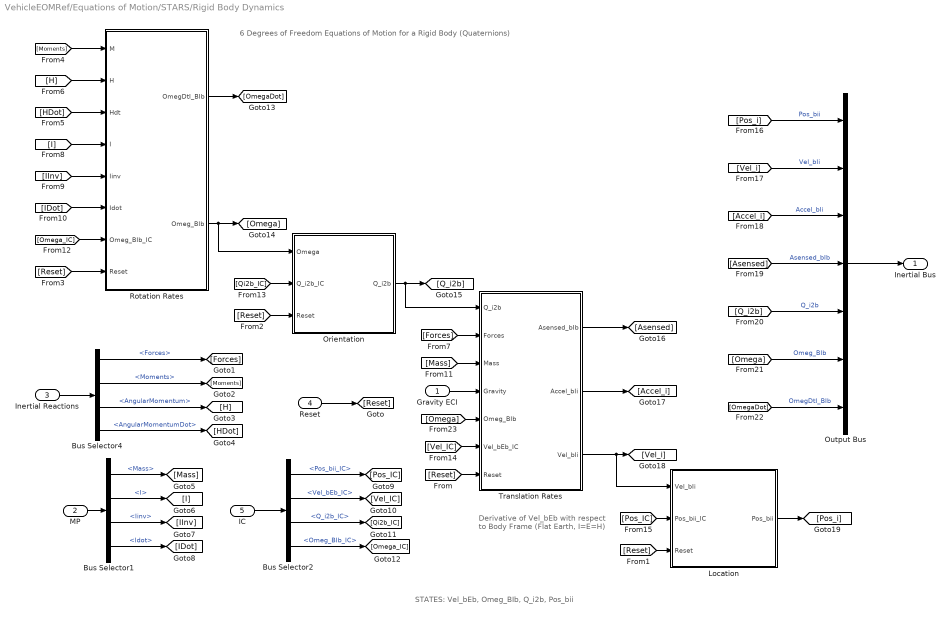
== system VehicleEOMRef/Equations of Motion/STARS/Rigid Body Dynamics ==
  note: 6 Degrees of Freedom Equations of Motion for a Rigid Body
      | (Quaternions)
  note: Derivative of Vel_bEb
      | with respect to Body Frame
      | (Flat Earth, I=E=H)
  note: STATES: Vel_bEb, Omeg_BIb, Q_i2b, Pos_bii
  Gravity ECI : Inport  PortDimensions=[3,1]
  MP : Inport  Port=2
  Inertial Reactions : Inport  Port=3
  Reset : Inport  Port=4
  IC : Inport  Port=5
  Bus Selector1 : BusSelector  OutputSignals=Mass,I,Iinv,Idot
  Bus Selector2 : BusSelector  OutputSignals=Pos_bii_IC,Vel_bEb_IC,Q_i2b_IC,Omeg_BIb_IC
  Bus Selector4 : BusSelector  OutputSignals=Forces,Moments,AngularMomentum,AngularMomentumDot
  Location : Subsystem
  Orientation : Subsystem
  Output Bus : BusCreator  Inputs=7
  Rotation Rates : Subsystem
  Translation Rates : Subsystem
  Inertial Bus : Outport
  wires:
  [Omega] -> Translation Rates/5(Omeg_BIb)
  [HDot] -> Rotation Rates/3(Hdt)
  [H] -> Rotation Rates/2(H)
  [Moments] -> Rotation Rates/1(M)
  Translation Rates/1(Asensed_bIb) -> [Asensed]
  Gravity ECI/1 -> Translation Rates/4(Gravity)
  Location/1(Pos_bii) -> [Pos_i]
  [Forces] -> Translation Rates/2(Forces)
  [Mass] -> Translation Rates/3(Mass)
  Translation Rates/2(Accel_bIi) -> [Accel_i]
  Translation Rates/3(Vel_bIi) -> Location/1(Vel_bIi), [Vel_i]
  Rotation Rates/2(Omeg_BIb) -> Orientation/1(Omega), [Omega]
  Rotation Rates/1(OmegDtI_BIb) -> [OmegaDot]
  Orientation/1(Q_i2b) -> Translation Rates/1(Q_i2b), [Q_i2b]
  [Reset] -> Translation Rates/7(Reset)
  [Reset] -> Location/3(Reset)
  [Reset] -> Orientation/3(Reset)
  [Reset] -> Rotation Rates/8(Reset)
  Reset/1 -> [Reset]
  Inertial Reactions/1 -> Bus Selector4/1
  Bus Selector4/1 -> [Forces]  "<Forces>"
  Bus Selector4/2 -> [Moments]  "<Moments>"
  Bus Selector4/3 -> [H]  "<AngularMomentum>"
  Bus Selector4/4 -> [HDot]  "<AngularMomentumDot>"
  MP/1 -> Bus Selector1/1
  Bus Selector1/1 -> [Mass]  "<Mass>"
  Bus Selector1/2 -> [I]  "<I>"
  Bus Selector1/3 -> [IInv]  "<Iinv>"
  Bus Selector1/4 -> [IDot]  "<Idot>"
  [I] -> Rotation Rates/4(I)
  [IInv] -> Rotation Rates/5(Iinv)
  [IDot] -> Rotation Rates/6(Idot)
  IC/1 -> Bus Selector2/1
  Bus Selector2/1 -> [Pos_IC]  "<Pos_bii_IC>"
  Bus Selector2/2 -> [Vel_IC]  "<Vel_bEb_IC>"
  Bus Selector2/3 -> [Qi2b_IC]  "<Q_i2b_IC>"
  Bus Selector2/4 -> [Omega_IC]  "<Omeg_BIb_IC>"
  [Omega_IC] -> Rotation Rates/7(Omeg_BIb_IC)
  [Qi2b_IC] -> Orientation/2(Q_i2b_IC)
  [Vel_IC] -> Translation Rates/6(Vel_bEb_IC)
  [Pos_IC] -> Location/2(Pos_bii_IC)
  [Pos_i] -> Output Bus/1  "Pos_bii"
  [Vel_i] -> Output Bus/2  "Vel_bIi"
  [Accel_i] -> Output Bus/3  "Accel_bIi"
  [Asensed] -> Output Bus/4  "Asensed_bIb"
  [Q_i2b] -> Output Bus/5  "Q_i2b"
  [Omega] -> Output Bus/6  "Omeg_BIb"
  [OmegaDot] -> Output Bus/7  "OmegDtI_BIb"
  Output Bus/1 -> Inertial Bus/1

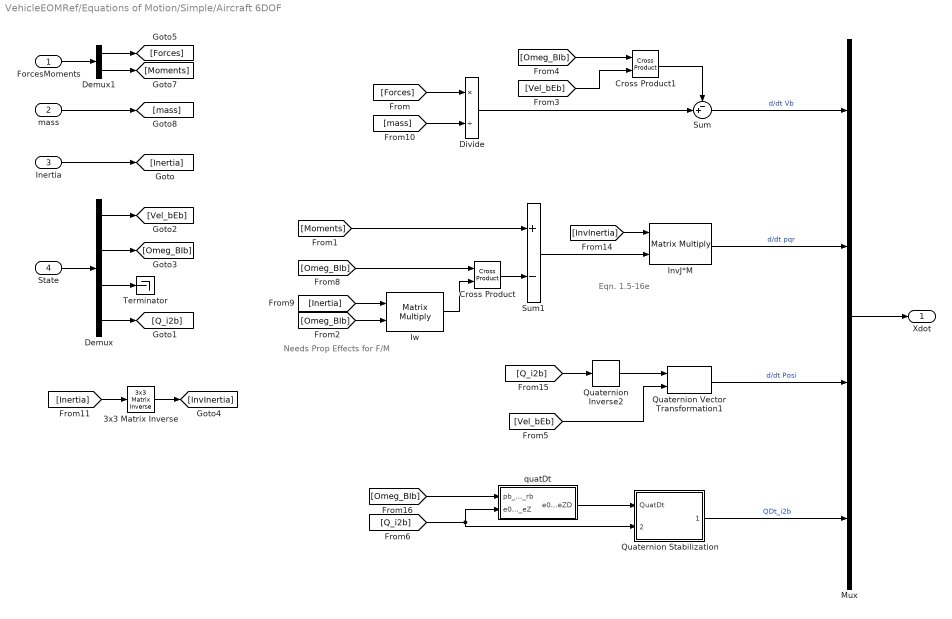
== system VehicleEOMRef/Equations of Motion/Simple/Aircraft 6DOF ==
  note: Eqn. 1.5-16e
  note: Needs Prop Effects for F/M
  ForcesMoments : Inport
  mass : Inport  Port=2
  Inertia : Inport  Port=3
  State : Inport  Port=4
  3x3 Matrix Inverse : starslibMathOperations/3x3 Matrix Inverse
  Cross Product : starslibMathOperations/Cross Product
  Cross Product1 : starslibMathOperations/Cross Product
  Demux : Demux  Outputs=[3 3 3 4]
  Demux1 : Demux  Outputs=[3 3]
  Divide : Product  Inputs=*/
  InvJ*M : Product  Multiplication=Matrix(*)
  Iw : Product  Multiplication=Matrix(*)
  Mux : Mux
  Quaternion Stabilization : Subsystem
  Quaternion Inverse2 : starslibMathOperations/Quaternion Inverse  n=0
  Quaternion Vector Transformation1 : starslibAxisTransformations/Quaternion Vector Transformation  n=0
  Sum : Sum  Inputs=-+|  SaturateOnIntegerOverflow=on
  Sum1 : Sum  Inputs=+-  SaturateOnIntegerOverflow=on
  Terminator : Terminator
  quatDt : Subsystem  mask(QuatDt){}
      mask help:
      | Calculates rate of change of orientation
      | quaternion (i.e. d{e0,eX,eY,eZ}/dt) (1/sec)
      | based on body axis rotational rates {p,q,r}
      | (rad/sec), & current orientation quaternion
      | {e0,eX,eY,eZ} (non-dimensional).
      mask Help:
      | <h4>Block Description</h4><p>
      | 
      | Calculates rate of change of orientation quaternion (i.e. d{e<sub>0</sub>,e<sub>X</sub>,e<sub>Y</sub>,e<sub>Z</sub>}/dt) (1/sec)
      | <br />based on body axis rotational rates {p,q,r} (rad/sec),
      | <br />&amp; current orientation quaternion {e<sub>0</sub>,e<sub>X</sub>,e<sub>Y</sub>,e<sub>Z</sub>} (non-dimensional).
      | 
      | </p><p>The block input and output contain more than one signal as described below.</p>
      | 
      | <table><thead><strong>Reference Documents</strong></thead>
      | <tr>
      | <td align="center" width="45">
      | <cite><strong>Review of Attitude Representations
      | <br />Used for Aircraft Kinematics</strong>
      | <br />Journal of Aircraft
      | <br />Vol. 38, No. 4, July-August 2001
      | 
      | <!---
      | <br />W.F. Phillips and C.E. Hailey
      | <br />Utah State University, Logan, UT  84322
      | <br />and
      | <br />G.A. Gebert
      | <br />Sverdrup Technology, Inc.
      | <br />Eglin AFB, FL 32542
      | --->
      | 
      | </cite></td>
      | <td width="5%"></td>
      | <td align="center" width="50%"><cite><strong>Recommended Practice for Atmospheric and
      | <br />Space Flight Vehicle Coordinate Systems</strong>
      | <br />ANSI&#47;AIAA   R-004-1992
      | <br />American National Standard Institute
      | <br />sponsored by
      | <br />American Institute of
      | <br />Aeronautics &amp; Astronautics</cite></td>
      | </tr>
      | <tr><td align="center" width="45%"><strong>Equation:
      | </strong> (31)</td>
      | <td width="5%"></td>
      | <td align="center" width="50%"><strong>
      | Sign convention from:</strong> (1.4.6)</td></tr>
      | </table>
      | 
      | <!---Implemented by David Christhilf
      |         Lockheed - Martin Engr. &amp; Sc. Co.
      |         Langley Program Office
      |         supporting NASA-Langley Research Center
      |         2002-08-21
      |         d.m.christhilf@larc.nasa.gov--->
      | 
      | <h4>Block Vector Input Port #1 - Body Axis Rotational Rates (rad/sec)</h4>
      | <table><tr>
      | <td><ul>
      |    <li>pb_rps</li>
      |    <li>qb_rps</li>
      |    <li>rb_rps</li>
      | </ul></td>
      | <td><dl><br />
      |    <dd>roll rate</dd>
      |    <dd>pitch rate</dd>
      |    <dd>yaw rate</dd>
      | </dl></td>
      | <td align="center"><dl><br />
      |    <dd>(+rt_wing_dn)</dd>
      |    <dd>(+nose_up)</dd>
      |    <dd>(+nose_rt)</dd>
      | </dl></td>
      | </tr></table>
      | 
      | <h4>Block Vector Input Port #2 - Orientation Quaternion (non-dimensional)</h4>
      | <ul>
      |    <li>e<sub>0</sub></li>
      |    <li>e<sub>X</sub></li>
      |    <li>e<sub>Y</sub></li>
      |    <li>e<sub>Z</sub></li>
      | </ul>
      | 
      | <h4>Block Vector Output - Time Derivative of Orientation Quaternion (1/sec)</h4>
      | <ul>
      |    <li>e0dt</li>
      |    <li>eXdt</li>
      |    <li>eYdt</li>
      |    <li>eZdt</li>
      | </ul>
      mask Display: disp('QuatDt')
  Xdot : Outport  VectorParamsAs1DForOutWhenUnconnected=off
  wires:
  Demux/3 -> Terminator/1
  [Vel_bEb] -> Quaternion Vector Transformation1/2
  Quaternion Vector Transformation1/1 -> Mux/3  "d/dt Posi"
  [Q_i2b] -> Quaternion Inverse2/1
  Quaternion Inverse2/1 -> Quaternion Vector Transformation1/1
  [Inertia] -> 3x3 Matrix Inverse/1
  [mass] -> Divide/2
  mass/1 -> [mass]
  Demux1/2 -> [Moments]
  Demux1/1 -> [Forces]
  ForcesMoments/1 -> Demux1/1
  Demux/4 -> [Q_i2b]
  Quaternion Stabilization/1(qdot out) -> Mux/4  "QDt_i2b"
  [Omeg_BIb] -> quatDt/1(pb_qb_rb)
  [Q_i2b] -> quatDt/2(e0_eX_eY_eZ), Quaternion Stabilization/2(Quat_i2b)
  quatDt/1(e0D_eXD_eYD_eZD) -> Quaternion Stabilization/1(QuatDt)
  Mux/1 -> Xdot/1
  Demux/2 -> [Omeg_BIb]
  Demux/1 -> [Vel_bEb]
  State/1 -> Demux/1
  Divide/1 -> Sum/2
  Cross Product1/1 -> Sum/1
  InvJ*M/1 -> Mux/2  "d/dt pqr"
  [InvInertia] -> InvJ*M/1
  Sum1/1 -> InvJ*M/2
  Cross Product/1 -> Sum1/2
  [Omeg_BIb] -> Cross Product/1
  Iw/1 -> Cross Product/2
  [Inertia] -> Iw/1
  [Omeg_BIb] -> Iw/2
  [Vel_bEb] -> Cross Product1/2
  [Omeg_BIb] -> Cross Product1/1
  [Moments] -> Sum1/1
  [Forces] -> Divide/1
  Sum/1 -> Mux/1  "d/dt Vb"
  3x3 Matrix Inverse/1 -> [InvInertia]
  Inertia/1 -> [Inertia]

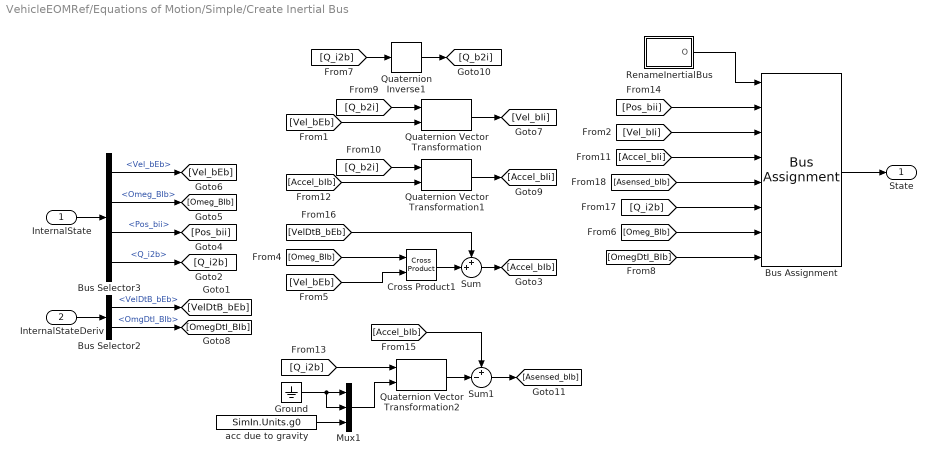
== system VehicleEOMRef/Equations of Motion/Simple/Create Inertial Bus ==
  InternalState : Inport
  InternalStateDeriv : Inport  Port=2
  Bus Assignment : BusAssignment  AssignedSignals=Pos_bii,Vel_bIi,Accel_bIi,Asensed_bIb,Q_i2b,Omeg_BIb,OmegDtI_BIb
  Bus Selector2 : BusSelector  OutputSignals=VelDtB_bEb,OmgDtI_BIb
  Bus Selector3 : BusSelector  OutputSignals=Vel_bEb,Omeg_BIb,Pos_bii,Q_i2b
  Cross Product1 : starslibMathOperations/Cross Product
  Ground : Ground
  Mux1 : Mux  Inputs=3
  Quaternion Inverse1 : starslibMathOperations/Quaternion Inverse  n=0
  Quaternion Vector Transformation : starslibAxisTransformations/Quaternion Vector Transformation  n=0
  Quaternion Vector Transformation1 : starslibAxisTransformations/Quaternion Vector Transformation  n=0
  Quaternion Vector Transformation2 : starslibAxisTransformations/Quaternion Vector Transformation  n=0
  RenameInertialBus : Subsystem
  Sum : Sum  Inputs=++|  SaturateOnIntegerOverflow=on
  Sum1 : Sum  Inputs=+-|  SaturateOnIntegerOverflow=on
  acc due to gravity : Constant  Value=SimIn.Units.g0
  State : Outport  VectorParamsAs1DForOutWhenUnconnected=off
  wires:
  Sum1/1 -> [Asensed_bIb]
  [Accel_bIb] -> Sum1/1
  Quaternion Vector Transformation2/1 -> Sum1/2
  [Q_i2b] -> Quaternion Vector Transformation2/1
  Mux1/1 -> Quaternion Vector Transformation2/2
  Ground/1 -> Mux1/1, Mux1/2
  acc due to gravity/1 -> Mux1/3
  [Accel_bIb] -> Quaternion Vector Transformation1/2
  Sum/1 -> [Accel_bIb]
  Cross Product1/1 -> Sum/2
  [VelDtB_bEb] -> Sum/1
  [Omeg_BIb] -> Cross Product1/1
  [Vel_bEb] -> Cross Product1/2
  [OmegDtI_BIb] -> Bus Assignment/8
  [Omeg_BIb] -> Bus Assignment/7
  [Q_i2b] -> Bus Assignment/6
  [Q_b2i] -> Quaternion Vector Transformation1/1
  Quaternion Vector Transformation1/1 -> [Accel_bIi]
  Quaternion Inverse1/1 -> [Q_b2i]
  [Q_i2b] -> Quaternion Inverse1/1
  Bus Selector2/2 -> [OmegDtI_BIb]  "<OmgDtI_BIb>"
  Bus Selector2/1 -> [VelDtB_bEb]  "<VelDtB_bEb>"
  Quaternion Vector Transformation/1 -> [Vel_bIi]
  [Vel_bEb] -> Quaternion Vector Transformation/2
  Bus Selector3/1 -> [Vel_bEb]  "<Vel_bEb>"
  Bus Selector3/2 -> [Omeg_BIb]  "<Omeg_BIb>"
  Bus Selector3/3 -> [Pos_bii]  "<Pos_bii>"
  Bus Selector3/4 -> [Q_i2b]  "<Q_i2b>"
  InternalState/1 -> Bus Selector3/1
  [Q_b2i] -> Quaternion Vector Transformation/1
  InternalStateDeriv/1 -> Bus Selector2/1
  Bus Assignment/1 -> State/1
  [Pos_bii] -> Bus Assignment/2
  [Accel_bIi] -> Bus Assignment/4
  [Asensed_bIb] -> Bus Assignment/5
  [Vel_bIi] -> Bus Assignment/3
  RenameInertialBus/1(O) -> Bus Assignment/1

== system VehicleEOMRef/Equations of Motion/Simple/Gravity ==
  State : Inport
  Bus Selector : BusSelector  OutputSignals=Q_i2b
  Display : Display
  Display1 : Display
  Display2 : Display
  Ground : Ground
  Ground1 : Ground
  Mux : Mux  Inputs=[3 3]
  Mux1 : Mux  Inputs=3
  Product1 : Product  RndMeth=Zero
  Quaternion Vector Transformation : starslibAxisTransformations/Quaternion Vector Transformation  n=0
  acc due to gravity : Constant  Value=SimIn.Units.g0
  mass : Constant  Value=SimIn.Model.mass
  FM : Outport  VectorParamsAs1DForOutWhenUnconnected=off
  wires:
  Bus Selector/1 -> Quaternion Vector Transformation/1, Display2/1  "<Q_i2b>"
  State/1 -> Bus Selector/1
  mass/1 -> Product1/1, Display/1
  Quaternion Vector Transformation/1 -> Mux/1
  Mux/1 -> FM/1
  Mux1/1 -> Quaternion Vector Transformation/2
  Ground/1 -> Mux1/1, Mux1/2
  Product1/1 -> Mux1/3
  Ground1/1 -> Mux/2
  acc due to gravity/1 -> Product1/2, Display1/1

== system VehicleEOMRef/Equations of Motion/Simple/State Labels ==
  I : Inport
  Bus Creator : BusCreator  Inputs=4
  Demux : Demux  Outputs=[3 3 3 4]
      settings: DisplayOption=none
  Reshape{1..3,5} (4 alike) : Reshape  OutputDimensionality=Column vector (2-D)
  O : Outport  VectorParamsAs1DForOutWhenUnconnected=off
  wires:
  Reshape5/1 -> Bus Creator/4  "Q_i2b"
  Reshape3/1 -> Bus Creator/3  "Pos_bii"
  Reshape2/1 -> Bus Creator/2  "Omeg_BIb"
  Reshape1/1 -> Bus Creator/1  "Vel_bEb"
  Demux/4 -> Reshape5/1  "Q_i2b"
  Demux/3 -> Reshape3/1  "Pos_bii"
  Demux/2 -> Reshape2/1  "Omeg_BIb"
  Demux/1 -> Reshape1/1  "Vel_bEb"
  Bus Creator/1 -> O/1
  I/1 -> Demux/1
